simulink model "mrefrobotarm"  (Simulink 8.1)
settings: Solver=ode45  SolverMode=SingleTasking  StartTime=0.0  StopTime=60  RelTol=1e-3  AbsTol=1e-6
undefined symbols (not defined in the file or in its folder): now, sfunxy2
libraries: neural x1
settings Model: Creator=matthew  LastModifiedBy=mbeale  ExtModeTrigMode=oneshot  ExtModeArmWhenConnect=off  TunableVars=prueba  TunableVarsStorageClass=Auto
settings DataIOCC: LimitDataPoints=off  SaveOutput=off  SignalLoggingName=sigsOut
settings OptimizationCC: BooleanDataType=off  InlineParams=on  InitFltsAndDblsToZero=on
settings DebuggingCC: SaveWithParameterizedLinksMsg=none  SignalResolutionControl=TryResolveAllWithWarning  SolverPrmCheckMsg=none  MultiTaskDSMMsg=warning  MultiTaskCondExecSysMsg=none  StrictBusMsg=None
settings HardwareCC: TargetUnknown=on
settings RTWCC: TemplateMakefile=grt_vc.tmf  IncludeERTFirstTime=on
settings GRTTargetCC: TargetFcnLib=ansi_tfl_tmw.mat

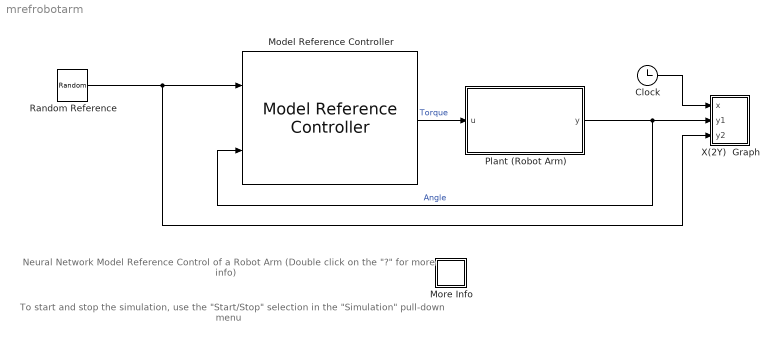
== system mrefrobotarm ==
  note: Neural Network Model Reference Control of a Robot Arm
      | (Double click on the "?" for more info)
  note: To start and stop the simulation, use the "Start/Stop"
      | selection in the "Simulation" pull-down menu
  Clock : Clock
  Model Reference Controller : neural/Control Systems/Model Reference Controller  Nrc=2  Nic=1  Njc=2  IW_y=[-0.069572273964750006 -0.50887837019159299;0.15074312774051651 0.11490189363692252;0.18140136858776268 0.37975663959876699;0.29517102307725995 -0.44709921582493495;-0.58875973816560423 -0.0401771725539046;0.72902870715668755 -0.58159644016547762;-0.79473114301336234 0.80685810458654827;-0.7203623145291248 1.750020475218397;0.32928031663047497 -0.34567654549749322;-0.68792644345580523 -1.22114357248857;-0.23114045526294194 0.52612028452189419;-0.078466033931512136 0.55740283259494039;0.5991557737260953 -0.0046772839951757239]  IW_u=[-0.28646849912653372;0.2082294676863414;-0.38700612728754513;-0.088356433428576742;-0.38246650005135652;-0.19979049829155976;0.12950350585422027;-0.076665336474221038;-0.26363250966352098;0.20162500315525875;0.15592324620945688;-0.28346970834751034;0.055516027366232526]  IW_r=[0.43133604056604929 2.2349303840625012;-0.25268785262535298 0.53956550757338506;-1.3942416031489167 1.6812760026264273;-2.2712469519952609 1.8940014540102785;0.62638823833708646 -1.5393599650914611;-1.3412735806395613 1.994061751122143;0.88233358538907281 -1.1149566012207308;1.2015877427658499 0.060457901863100086;1.3973493005875692 -1.2246446473460524;-1.1621604385833166 -1.1103119260029528;-1.7049791456903904 0.3100076441017976;2.1148038096378441 1.3849513797060495;-0.94244119059308828 1.6273823577565985]  B1_c=[2.5275336083252959;-2.015153508209353;-1.573574939030099;0.24807575673883855;0.72804063587227263;-0.15009860896928837;-0.14566022969189182;-0.14503306001354413;0.80257458525071157;-2.3204357652991572;-1.7091111210606085;-2.1755082369914769;2.3060895543527407]  B2_c=-0.89128704544185799  LW_c=[0.0090810097275292444 1.016994132671448 -0.57703994488362598 -1.4828532318010392 0.21544013872474743 -2.0819490128456084 1.951101458107841 2.2265872491488485 -0.20951152443698737 -2.4183248929210941 -0.17557803620122728 0.4111829140769851 -0.13651025081277837]  retraining_c=30  max_i_int=2  min_i_int=0.1  max_r_int=2  min_r_int=0.1  Ts=0.05  S1=10  Ni=2  Nj=2  sim_file=robotarm  trainfun=trainlm  Use_validation=1  Use_Testing=1  Use_Inc_training=0  Use_previous_weights=1  max_i=15  min_i=-15  max_r=0.7  min_r=-0.7  sam_training=10000  sam_training_c=6000  epochs=300  epochs_c=10  minp=-14.938368446677966  maxp=14.990917500914531  mint=-3.3006125056148323  maxt=3.2985736367119713  Normalize=0  IW=[0.67556972299583085 -0.69678512012524063;0.00091251541328585956 -0.0027081486615356675;0.00020438440527543628 0.00019904673243416438;0.00049656346445165877 0.0004751589166608323;0.83784411703306994 -0.26889964997200294;-0.00019020895770413364 -0.00011909258917915059;-0.40317423125635427 0.4194745680490527;-0.57818696835623018 0.57975674359031992;-0.00022043349689196401 -0.00021518711933560483;-0.00022005213616311755 -0.00014885817639699326]  LW1_2=[1.2764115081604008 -1.3654567744259543;0.89310137588971361 1.0042430979155006;0.33273669122142152 -0.15270262190099879;0.71703040374417737 -0.36195588775915477;-2.5505602345955283 -4.1931013065877298;-0.48162311647991762 0.1228304948598478;1.5080087551662273 -1.7803806270961875;0.58957956932235933 -0.1379494539478418;-0.35268820684492125 0.16442179826947986;-0.49711480585257867 0.14758471020788191]  LW2_1=[-1.3652007830674679e-006 -0.0002723650242372647 4.3375977757897157 0.38766138633249286 1.2167137492000295e-006 2.7535219948226088 1.2897509057532762e-006 -1.2811132141620941e-006 -4.4162135512266767 -2.9235276934566996]  B1=[8.3454601861727848;-1.7488652958811703;0.66134602652445429;1.9828413629191783;2.8470577972675652;0.0013587107297852578;-3.0111623514274384;-1.3201798813874432;0.88505814110298575;0.0084913784378921556]  B2=0.26583865321126832  S1c=13  Limit_output=1  min_output=-3.1  max_output=3.1  Ref_file=robotref
  More Info : Subsystem
      mask Display: disp('?')
  Plant (Robot Arm) : Subsystem
      mask Display: plot([-10],[0],[10],[0],[-2 -2 2 2 -2],[5 4 4 5 5],[0 3],[4.5 0.5])
  Random Reference : UniformRandomNumber  Minimum=-0.5  Maximum=0.5  Seed=round(now)  SampleTime=10
  X(2Y)  Graph : Subsystem  LoadFcn=sfunxy2([],[],[],'LoadBlock')  StartFcn=sfunxy2([],[],[],'Start')  StopFcn=sfunxy2([],[],[],'Stop')  mask(X(2Y) scope.){xmin=0, xmax=5, ymin=-1, ymax=1, st=-1}
      mask prompts: xmin "x-min:"; xmax "x-max:"; ymin "y-min:"; ymax "y-max:"; st "Sample time:"
      mask help: X(2Y) scope using MATLAB graph window. First input is used as time base. Enter plotting ranges.
      settings: CopyFcn=sfunxy2([],[],[],'CopyBlock')  DeleteFcn=sfunxy2([],[],[],'DeleteBlock')  NameChangeFcn=sfunxy2([],[],[],'NameChange')
      mask Help: This block can be used to explore limit cycles. Look at the function sfunxy.m to see how it works.
      mask Display: plot([.05 .95 .95 .05 .05],[.45 .45 .95 .95 .45], 0.5+cos(0:0.1:2*pi)*0.3,0.7+sin(0:0.1:2*pi)*0.2)
  wires:
  Plant (Robot Arm)/1(y) -> X(2Y)  Graph/2(y1), Model Reference Controller/2  "Angle"
  Model Reference Controller/1 -> Plant (Robot Arm)/1(u)  "Torque"
  Clock/1 -> X(2Y)  Graph/1(x)
  Random Reference/1 -> X(2Y)  Graph/3(y2), Model Reference Controller/1

== system mrefrobotarm/More Info ==
  note: This system simulates model reference control
      | of a single-link robot arm.
  note: Double-click on the Model Reference Controller block
      | to train the neural network controller and plant model.
  note: For more information on what the controller
      | does, look under the mask of the Model Reference
      | Controller block.

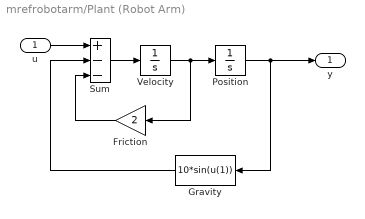
== system mrefrobotarm/Plant (Robot Arm) ==
  u : Inport
  Friction : Gain  Gain=2  SaturateOnIntegerOverflow=on  OutDataTypeStr=Inherit: Same as input  ParamDataTypeStr=Inherit: Same as input
  Gravity : Fcn  Expr=10*sin(u(1))
  Position : Integrator  ZeroCross=off
  Sum : Sum  Inputs=+--  SaturateOnIntegerOverflow=on  InputSameDT=on  OutDataTypeStr=Inherit: Same as first input
  Velocity : Integrator  ZeroCross=off
  y : Outport
  wires:
  Position/1 -> y/1, Gravity/1
  u/1 -> Sum/1
  Sum/1 -> Velocity/1
  Gravity/1 -> Sum/2
  Velocity/1 -> Position/1, Friction/1
  Friction/1 -> Sum/3

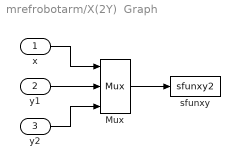
== system mrefrobotarm/X(2Y)  Graph ==
  x : Inport
  y1 : Inport  Port=2
  y2 : Inport  Port=3
  Mux : Mux  Inputs=3
  sfunxy : S-Function  FunctionName=sfunxy2  Parameters=[xmin xmax ymin ymax], st  EnableBusSupport=off
  wires:
  y2/1 -> Mux/3
  y1/1 -> Mux/2
  x/1 -> Mux/1
  Mux/1 -> sfunxy/1
